simulink model "weather_task"  (Simulink 3.00)
undefined symbols (not defined in the file): application, json, weather
libraries: stringlib x3, mathlib x1, speclib x1

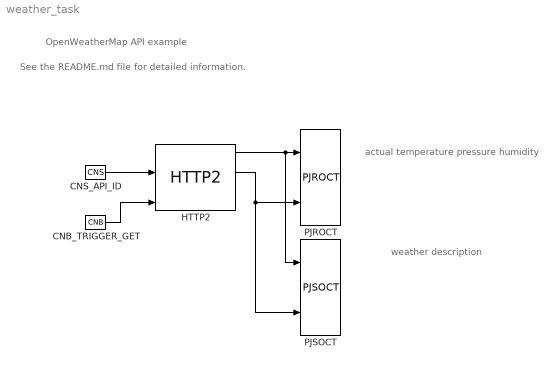
== system weather_task ==
  note: See the README.md file for detailed information.
  note: OpenWeatherMap API example
  note: weather
      | description
  note: actual temperature
      | pressure
      | humidity
  CNB_TRIGGER_GET : mathlib/CNB  YCN=off
  CNS_API_ID : stringlib/CNS  scv=YourAPIkey  nmax=0
  HTTP2 : speclib/HTTP2  url=http://api.openweathermap.org/data/2.5/weather?q=Pilsen&units=metric&appid=  method=1: GET  VERIFY=off  postmime=application/json  acceptmime=application/json  timeout=5  BLOCKING=off  nmax=0  postmax=256  datamax=1024
  PJROCT : stringlib/PJROCT  name1=main.temp  name2=main.pressure  name3=main.humidity  name4=main.sea_level  nmax=0  yerr=0.0000000000E+000
  PJSOCT : stringlib/PJSOCT  name1=weather[0].main  name2=weather[0].description  nmax=0
  wires:
  CNB_TRIGGER_GET/1 -> HTTP2/4
  CNS_API_ID/1 -> HTTP2/2
  HTTP2/1 -> PJROCT/1, PJSOCT/1
  HTTP2/3 -> PJROCT/2, PJSOCT/2
